simulink library "MISSILE_GUIDANCE_LIB2"  (R2025b)
settings: Solver=VariableStepAuto  StartTime=0.0  StopTime=10.0  RelTol=1e-3
undefined symbols (not defined in the file or in its folder): accelerationL0, angularPoseL0, angularRateL0, B2D, Continuous, ddLambda, dLambda, dRange, epsMEAS_D, L02B, Lambda, positionL0, psiDotCmd, psiMeas, Range, rangeDotMEAS_D, rangeMEAS_D, t_go, t_sim, targetEps_D, targetRelPos_B, targetRelPos_D, targetRelPos_L0, targetRelVel_L0, targetValid, thetaDotCmd, thetaMeas, Time, timeOfMeas, velocityL0, wAfterStabTF, wCmd_Rtn
libraries: $bdroot x27, simulink x8, simulink_extras x6, matrix_library x3, Missile_Guidance_LIB x1, ctrlSharedLib x1
(part 1 of 2)
settings Model: Creator=leoni  LastModifiedBy=Leonid
settings RTWCC: GPUComputeCapability=3.5

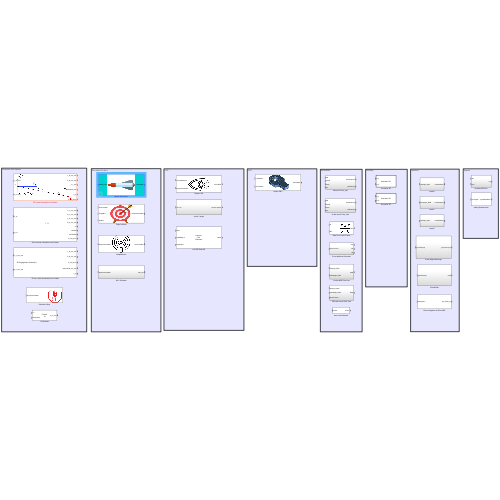
[thumbnail: Simulink's stored preview of the top-level diagram]
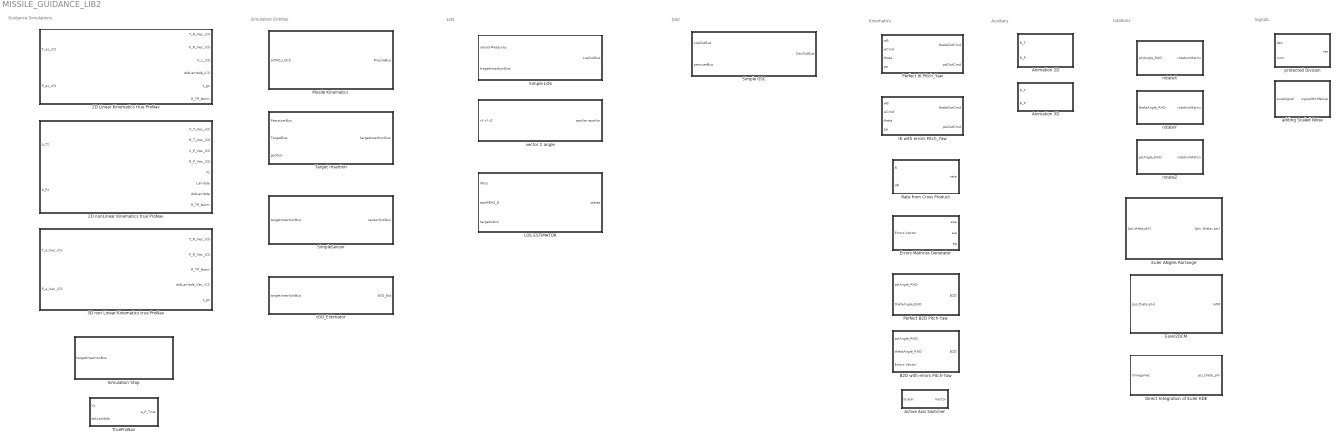
== system MISSILE_GUIDANCE_LIB2 ==
  note: Signals
  note: Auxiliary
  note: LOS
  note: GSC
  note: Simulation Entities
  note: rotations
  note: Kinematics
  note: Guidance Simulations
  2D Linear Kinematics true ProNav : Subsystem  mask{T_Vx0_iCS=-300, T_R0_Vec_iCS=[13000;0], P_Vx0_pCS=1000, P_R0_Vec_iCS=[0;0], HE=-20}
      mask prompts: T_Vx0_iCS "Target Horizontal Velocity [m/s]"; T_R0_Vec_iCS "Initial Target Position Vector [m]"; P_Vx0_pCS "Persuer velocity [m/s]"; P_R0_Vec_iCS "Initial Persuer Position Vector [m]"; HE "Persuer Heading Error Angle [deg]"
      mask DialogControl TargetGroup Prompt: Target Properties
      mask DialogControl PersuerGroup Prompt: Persuer Properties
      mask Display: image('Linearized 2D proNav Guidance.png');
  2D nonLinear Kinematics true ProNav : Subsystem  mask{V_T=300, R_Tx_0=1000, R_Tz_0=10, beta_0=rad2deg(10e-3), V_P=0, R_Px_0=0, R_Pz_0=0, gamma_0=0}
      mask prompts: V_T "Target Velocity [m/s]"; R_Tx_0 "Initial Target Position x [m]"; R_Tz_0 "Initial Target Position z [m]"; beta_0 "Initial Target Angle[deg]"; V_P "Persuer Velocity [m/s]"; R_Px_0 "Initial Pursuer Position x [m]"; R_Pz_0 "Initial Pursuer Position z [m]"; gamma_0 "Initial Pursuer Flight Path Angle[deg]"
      mask DialogControl TargetGroup Prompt: Target Properties
      mask DialogControl PursuerGroup Prompt: Pursuer properties
      mask Display: image('Collision_Course_Kinematics_2D.jpg');
  3D non Linear Kinematics true ProNav : Subsystem  mask{T_V0_Vec_iCS=[300*cos(10e-3);0;300*sin(10e-3)], T_R0_Vec_iCS=[-1000;0;0], P_V0_Vec_iCS=[0;0;0], P_R0_Vec_iCS=[0;0;0]}
      mask prompts: T_V0_Vec_iCS "Target Initial Velocity Vector [m/s]"; T_R0_Vec_iCS "Initial Target Position Vector [m]"; P_V0_Vec_iCS "Persuer Initial Velocity vector [m/s]"; P_R0_Vec_iCS "Initial Persuer Position Vector [m]"
      mask init:
      | if ~exist('Missile_Guidance_Bus_Load_Ok', 'var')
      | run Missile_Guidance_Buses.m
      | assignin('base', 'Missile_Guidance_Bus_Load_Ok', true);
      | fprintf('---- Missile Guidance Buses Loaded Ok ---- \n');
      | 
      | end
      mask DialogControl TargetGroup Prompt: Target Properties
      mask DialogControl PersuerGroup Prompt: Persuer Properties
      mask Display: text(0.05, 0.5, '3D Engagement Kinematics');
  Active Axis Switcher : Subsystem  mask{activeAxis=P motion}
      mask prompts: activeAxis "Base Sine Wave Selector"
      mask TypeOptions activeAxis: P motion | Q motion | R motion
  Animation 2D : MATLAB Function  TreatAsAtomicUnit=on  SystemSampleTime=0.1  mask{xlimVec=[-100 1100], ylimVec=[-20 20]}
      mask prompts: xlimVec "xlim [m]"; ylimVec "ylim [m]"
      mask init:
      | figure('Name','Simulation')
      |     close all;
      |     clf;
      |     plot([],[]); hold on;
      | 
      | 
      |     xlim(xlimVec)
      |     ylim(ylimVec)
      |     % axis equal
      |     grid minor
      |     xlabel('Xaxis [m]')
      |     ylabel('Zaxis [m]')
  Animation 3D : MATLAB Function  TreatAsAtomicUnit=on  SystemSampleTime=0.1  mask{xlimVec=[-1000 20], ylimVec=[-10 10], zlimVec=[-20 20]}
      mask prompts: xlimVec "xlim [m]"; ylimVec "ylim [m]"; zlimVec "zlim [m]"
      mask init:
      | figure('Name','Simulation3D')
      |     close all;
      |     clf;
      |     plot3([0],[0],[0]); hold on;
      | 
      | 
      |     xlim(xlimVec)
      |     ylim(ylimVec)
      |     zlim(zlimVec)
      |     % axis equal
      |     grid minor
      |     xlabel('Xaxis [m]')
      |     ylabel('Yaxis [m]')
      |     zlabel('Zaxis [m]')
  B2D with errors Pitch-Yaw : Subsystem
  Direct Integration of Euler KDE : Subsystem  mask{psi0_theta0_phi0=[0;0;0]}
      mask prompts: psi0_theta0_phi0 "Initial Pose Angles [psi0;theta0;phi0] [deg]"
      mask DialogControl ic1 Prompt: Initial Conditions
  Errors Matrices Generator : Subsystem
  Euler ANgles Rarrange : Subsystem
  Euler2DCM : Subsystem
  IK with errors Pitch_Yaw : Subsystem
  LOS ESTIMATOR : Subsystem  mask{Q=0.1, R=0.1}
      mask prompts: Q "Q - value"; R "R - value"
      mask DialogControl ParameterGroupVar Prompt: Esimator Parameters
      mask Display: disp('Lambda \n Dot \n Estimator');
  Missile Kinematics : Subsystem  mask{psi0_theta0_phi0=[0;0;0], vX0=0, r0=[0;0;0], tau_X=0, tau_YZ=0}
      mask prompts: psi0_theta0_phi0 "Initial [psi0;theta0;phi0] Angles [deg]"; vX0 "Initial Velocity missile X [m/s]"; r0 "Initial Position L0 [m]"; tau_X "Longitudinal time constant [s]"; tau_YZ "Lateral time constant [s]"
      mask DialogControl ParameterGroupVar Prompt: Initial Conditions
      mask DialogControl Container3 Prompt: Psuedo Pilot
      mask Display: image('missile.png');
  Perfect B2D Pitch-Yaw : Subsystem
  Perfect IK Pitch_Yaw : Subsystem
  Rate from Cross Product : Subsystem
      mask Display: image('Rate_From_Cross_Product.png');
  Simple GSC : Subsystem  mask{theta0=0, psi0=0, fRATE=0, zetaRATE=0, f_clock_GSC=1800, enErrors=on, errorsVec=zeros(9,1), Jo_kgmm=0, Ji_kgmm=0, Icmd_MAX=0, Kt_mNm=0}
      mask prompts: theta0 "Initial Pitch Angle [deg]"; psi0 "Initial yaw Angle [deg]"; fRATE "Rate Controller fBW [Hz]"; zetaRATE "Rate Controller Zeta"; f_clock_GSC "GSC Working Freq [Hz]"; enErrors "Enable Errors"; errorsVec "Errors Vector - X (terms)"; Jo_kgmm "Outer Inertia [kgmm^2]"; Ji_kgmm "Inner Inertia [kgmm^2]"; Icmd_MAX "Current Limit [A]"; Kt_mNm "Motor Constant [mNm/A]"
      mask DialogControl ParameterGroupVar Prompt: Initial Conditions
      mask DialogControl Container3 Prompt: Rate Controller
      mask DialogControl Container4 Prompt: RT parameters
      mask DialogControl Container5 Prompt: Installation Errors
      mask DialogControl Container6 Prompt: Mass Params
      mask DialogControl Container7 Prompt: Current Params
      mask Display: image('GIMBALS.png');
  Simple LOS : Subsystem  mask{kLOS=0, f_clock_LOS=600, perfectPoint=on, perfectTrack=on}
      mask prompts: kLOS "Track Loop Gain"; f_clock_LOS "Los Working Freq [Hz]"; perfectPoint "Is Perfect Point Mode ?"; perfectTrack "Is Perfect Tack Mode ?"
      mask DialogControl ParameterGroupVar Prompt: Controllers
      mask DialogControl Container3 Prompt: RT
      mask DialogControl Container4 Prompt: Assumptions
      mask Display: image('LOS.png');
  SimpleSensor : Subsystem  mask{halfFov=0, epsNoise=0, rangeNoise=0, rangeDotNoise=0, f_clock_SENS=100, tLatency=10}
      mask prompts: halfFov "Half Sensors FOV [deg]"; epsNoise "Epsilon Noise [rad]"; rangeNoise "Range Noise [m]"; rangeDotNoise "Dopler Noise [m/s]"; f_clock_SENS "Reporting Freq. [Hz]"; tLatency "Reporting Latency [ms]"
      mask DialogControl ParameterGroupVar Prompt: Sensor Parameters
      mask DialogControl Container3 Prompt: RT Parameters
      mask Display: image('Sensor.png');
  Simulation Stop : Subsystem  mask{tGO_Limit=0}
      mask prompts: tGO_Limit "Maximum TGO Value [s]"
      mask Display: image('STOP.png');
  Target Insertion : Subsystem
      mask Display: image('Target.png');
  TrueProNav : Subsystem  mask{N=3}
      mask prompts: N "ProNav Coefficient - N"
      mask Display: disp('ProNav\n N');
  adding Scaled Noise : Subsystem  mask{noiseProc=0}
      mask prompts: noiseProc "Noise [%] from Signal"
  protected Division : Subsystem
  rotateX : Subsystem
  rotateY : Subsystem
  rotateZ : Subsystem
  tGO_Estimator : Subsystem
  vector 2 angle : Subsystem

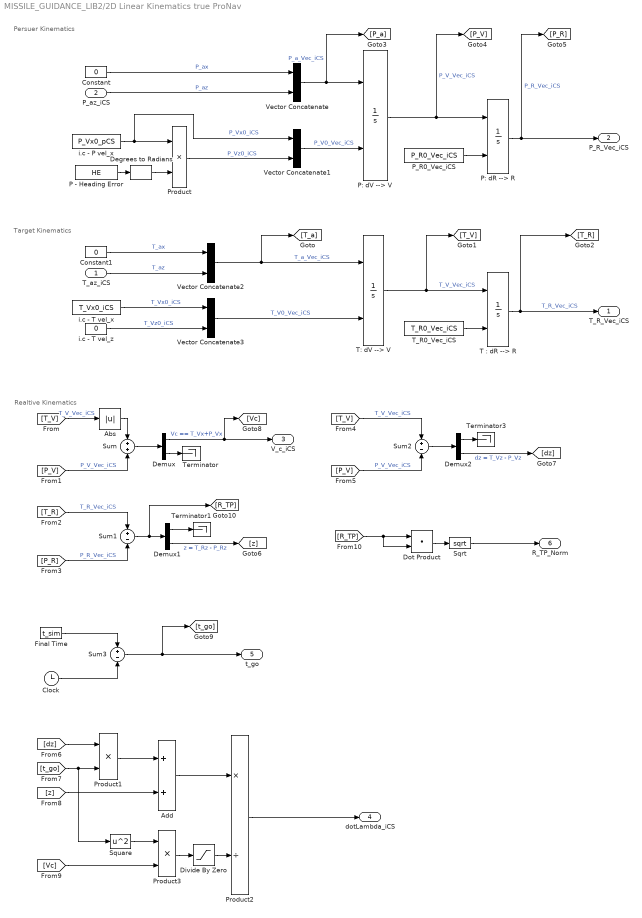
== system MISSILE_GUIDANCE_LIB2/2D Linear Kinematics true ProNav ==
  note: Persuer Kinematics
  note: Target Kinematics
  note: Realtive Kinematics
  T_az_iCS : Inport
  P_az_iCS : Inport  Port=2
  Abs : Abs  SaturateOnIntegerOverflow=off
  Add : Sum
  Clock : Clock
  Constant : Constant  Value=0
  Constant1 : Constant  Value=0
  Degrees to Radians : simulink_extras/Transformations/Degrees to Radians
  Demux : Demux  Outputs=2
  Demux1 : Demux  Outputs=2
  Demux2 : Demux  Outputs=2
  Divide By Zero : Saturate  UpperLimit=Inf  LowerLimit=1e-9
  Dot Product : DotProduct  OutDataTypeStr=Inherit: Inherit via internal rule
  Final Time : Constant  Value=t_sim
  P - Heading Error : Constant  Value=HE
  P: dR --> R : Integrator  InitialConditionSource=external
  P: dV --> V : Integrator  InitialConditionSource=external
  P_R0_Vec_iCS : Constant  Value=P_R0_Vec_iCS
  Product : Product
  Product1 : Product
  Product2 : Product  Inputs=*/
  Product3 : Product
  Sqrt : Sqrt
  Square : Math  Operator=square
  Sum : Sum  Inputs=+|+
  Sum1 : Sum  Inputs=+|-
  Sum2 : Sum  Inputs=+|-
  Sum3 : Sum  Inputs=+|-
  "T : dR --> R" : Integrator  InitialConditionSource=external
  T: dV --> V : Integrator  InitialConditionSource=external
  T_R0_Vec_iCS : Constant  Value=T_R0_Vec_iCS
  Terminator : Terminator
  Terminator1 : Terminator
  Terminator3 : Terminator
  Vector Concatenate{,1..3} (4 alike) : Concatenate  Mode=Multidimensional array
  i.c - P vel_x : Constant  Value=P_Vx0_pCS
  i.c - T vel_x : Constant  Value=T_Vx0_iCS
  i.c - T vel_z : Constant  Value=0
  T_R_Vec_iCS : Outport
  P_R_Vec_iCS : Outport  Port=2
  V_c_iCS : Outport  Port=3
  dotLambda_iCS : Outport  Port=4
  t_go : Outport  Port=5
  R_TP_Norm : Outport  Port=6
  wires:
  Divide By Zero/1 -> Product2/2
  Abs/1 -> Sum/1
  Sqrt/1 -> R_TP_Norm/1
  Dot Product/1 -> Sqrt/1
  [R_TP] -> Dot Product/1, Dot Product/2
  Product2/1 -> dotLambda_iCS/1
  Product3/1 -> Divide By Zero/1
  Square/1 -> Product3/1
  [Vc] -> Product3/2
  Add/1 -> Product2/1
  [z] -> Add/2
  Product1/1 -> Add/1
  [dz] -> Product1/1
  [t_go] -> Product1/2, Square/1
  Sum3/1 -> [t_go], t_go/1
  Final Time/1 -> Sum3/1
  Clock/1 -> Sum3/2
  [P_V] -> Sum2/2  "P_V_Vec_iCS"
  [T_V] -> Sum2/1  "T_V_Vec_iCS"
  Sum2/1 -> Demux2/1
  Demux2/1 -> Terminator3/1
  Demux2/2 -> [dz]  "dz = T_Vz - P_Vz"
  Demux1/2 -> [z]  "z = T_Rz - P_Rz"
  Demux1/1 -> Terminator1/1
  Sum1/1 -> Demux1/1, [R_TP]
  [P_R] -> Sum1/2  "P_R_Vec_iCS"
  [T_R] -> Sum1/1  "T_R_Vec_iCS"
  Demux/1 -> V_c_iCS/1, [Vc]  "Vc == T_Vx+P_Vx"
  Demux/2 -> Terminator/1
  Sum/1 -> Demux/1
  [P_V] -> Sum/2  "P_V_Vec_iCS"
  [T_V] -> Abs/1  "T_V_Vec_iCS"
  "T : dR --> R"/1 -> T_R_Vec_iCS/1, [T_R]  "T_R_Vec_iCS"
  T_R0_Vec_iCS/1 -> "T : dR --> R"/2
  Degrees to Radians/1 -> Product/2
  T: dV --> V/1 -> "T : dR --> R"/1, [T_V]  "T_V_Vec_iCS"
  Vector Concatenate3/1 -> T: dV --> V/2  "T_V0_Vec_iCS"
  i.c - T vel_z/1 -> Vector Concatenate3/2  "T_Vz0_iCS"
  i.c - T vel_x/1 -> Vector Concatenate3/1  "T_Vx0_iCS"
  Vector Concatenate2/1 -> T: dV --> V/1, [T_a]  "T_a_Vec_iCS"
  Constant1/1 -> Vector Concatenate2/1  "T_ax"
  P: dR --> R/1 -> P_R_Vec_iCS/1, [P_R]  "P_R_Vec_iCS"
  Vector Concatenate1/1 -> P: dV --> V/2  "P_V0_Vec_iCS"
  Vector Concatenate/1 -> P: dV --> V/1, [P_a]  "P_a_Vec_iCS"
  Constant/1 -> Vector Concatenate/1  "P_ax"
  Product/1 -> Vector Concatenate1/2  "P_Vz0_iCS"
  P - Heading Error/1 -> Degrees to Radians/1
  P_R0_Vec_iCS/1 -> P: dR --> R/2
  P: dV --> V/1 -> P: dR --> R/1, [P_V]  "P_V_Vec_iCS"
  i.c - P vel_x/1 -> Product/1, Vector Concatenate1/1  "P_Vx0_iCS"
  P_az_iCS/1 -> Vector Concatenate/2  "P_az"
  T_az_iCS/1 -> Vector Concatenate2/2  "T_az"

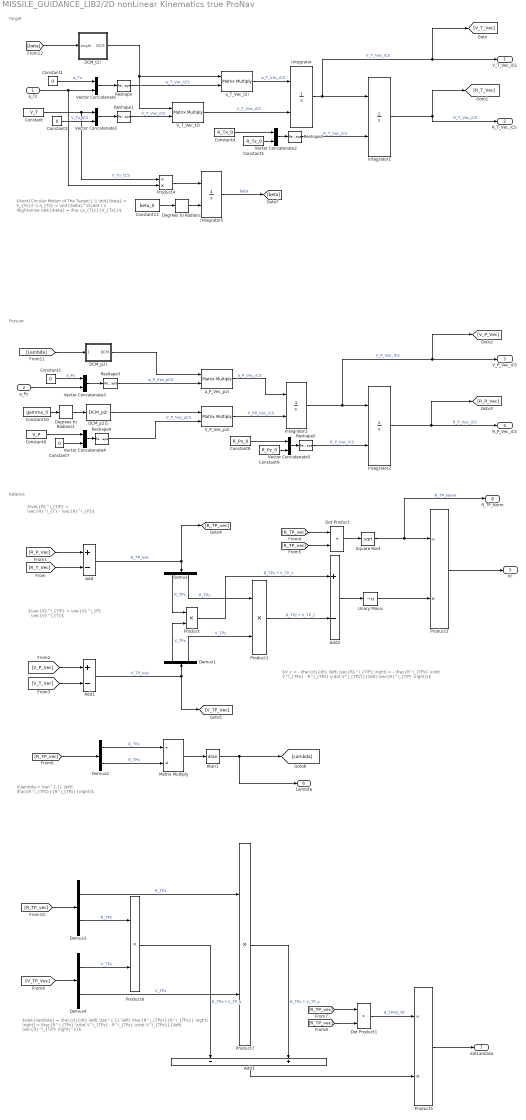
== system MISSILE_GUIDANCE_LIB2/2D nonLinear Kinematics true ProNav ==
  note: $\dot{\lambda} = \frac{d}{dt} \left[ \tan^{-1} \left( \frac{R^i_{TPz}}{R^i_{TPx}} \right) \right] = \frac{R^i_{TPx} \cdot V^i_{TPz} - R^i_{TPz} \cdot V^i_{TPx}}{\left| \vec{R}^i_{T/P} \right|^2}$
  note: $\vec{V}^i_{T/P} = \vec{V}^i_{P} - \vec{V}^i_{T}$
  note: Persuer
  note: Target
  note: Relative
  note: $\vec{R}^i_{T/P} = \vec{R}^i_{T} - \vec{R}^i_{P}$
  note: $V_c = - \frac{d}{dt} \left| \vec{R}^i_{T/P} \right| = - \frac{R^i_{TPx} \cdot V^i_{TPx} - R^i_{TPz} \cdot V^i_{TPz}}{\left| \vec{R}^i_{T/P} \right|}$
  note: $\lambda = \tan^{-1} \left( \frac{R^i_{TPz}}{R^i_{TPx}}\right)$
  note: $\text{Circular Motion of The Target:} \\ \dot{\beta} = V_{Tx}/r \\ a_{Tz} = \dot{\beta}^2\cdot r \\ \Rightarrow \dot{\beta} = \frac{a_{Tz}}{V_{Tx}}$
  a_Tz : Inport
  a_Pz : Inport  Port=2
  Add : Sum  Inputs=+-
  Add1 : Sum  Inputs=+-
  Add2 : Sum  Inputs=+-
  Add3 : Sum  Inputs=-+
  Atan1 : Trigonometry  Operator=atan
  Constant : Constant  Value=V_T
  Constant{1..3,7} (4 alike) : Constant  Value=0
  Constant10 : Constant  Value=gamma_0
  Constant11 : Constant  Value=beta_0
  Constant4 : Constant  Value=R_Tx_0
  Constant5 : Constant  Value=R_Tz_0
  Constant6 : Constant  Value=V_P
  Constant8 : Constant  Value=R_Px_0
  Constant9 : Constant  Value=R_Pz_0
  DCM_p2i : Subsystem
  DCM_p2i1 : Missile_Guidance_LIB/2D nonLinear Kinematics true ProNav/DCM_p2i  SystemSampleTime=-1  VariantActivationTime=update diagram  AllowFlexibleInterface=on  Latency=0  AutoFrameSizeCalculation=off
  DCM_t2i : Subsystem
  Degrees to Radians : simulink_extras/Transformations/Degrees to Radians
  Degrees to Radians1 : simulink_extras/Transformations/Degrees to Radians
  Demux{,1..4} (5 alike) : Demux  Outputs=2
  Dot Product : DotProduct  OutDataTypeStr=Inherit: Inherit via internal rule
  Dot Product1 : DotProduct  OutDataTypeStr=Inherit: Inherit via internal rule
  Integrator{,1..3,5} (5 alike) : Integrator  InitialConditionSource=external
  Matrix Multiply : Product  Inputs=/*
  Product{,1,6..7} (4 alike) : Product
  Product2 : Product  Inputs=/*
  Product4 : Product  Inputs=/*
  Product5 : Product  Inputs=/*
  Reshape{,1..5} (6 alike) : Reshape  OutputDimensionality=Column vector (2-D)
  Square Root : Sqrt
  Unary Minus : UnaryMinus
  V_P_Vec_p2i : Product  Multiplication=Matrix(*)
  V_T_Vec_t2i : Product  Multiplication=Matrix(*)
  Vector Concatenate{,1..5} (6 alike) : Concatenate
  a_P_Vec_p2i : Product  Multiplication=Matrix(*)
  a_T_Vec_t2i : Product  Multiplication=Matrix(*)
  V_T_Vec_iCS : Outport
  R_T_Vec_iCS : Outport  Port=2
  V_P_Vec_iCS : Outport  Port=3
  R_P_Vec_iCS : Outport  Port=4
  Vc : Outport  Port=5
  Lambda : Outport  Port=6
  dotLambda : Outport  Port=7
  R_TP_Norm : Outport  Port=8
  wires:
  Atan1/1 -> [Lambda], Lambda/1
  Matrix Multiply/1 -> Atan1/1
  Degrees to Radians1/1 -> DCM_p2i1/1
  DCM_p2i1/1 -> V_P_Vec_p2i/1
  Constant10/1 -> Degrees to Radians1/1
  V_P_Vec_p2i/1 -> Integrator2/2  "V_P0_Vec_iCS"
  Degrees to Radians/1 -> Integrator5/2
  V_T_Vec_t2i/1 -> Integrator/2  "V_T_Vec_iCS"
  Integrator5/1 -> [beta]  "beta"
  Constant11/1 -> Degrees to Radians/1
  Product4/1 -> Integrator5/1
  Product7/1 -> Add3/2  "R_TPx * V_TP_z"
  Product6/1 -> Add3/1  "R_TPz * V_TP_x"
  [R_TP_vec] -> Demux3/1
  [V_TP_Vec] -> Demux4/1
  Demux4/1 -> Product6/2  "V_TPx"
  Demux3/2 -> Product6/1  "R_TPz"
  Demux3/1 -> Product7/1  "R_TPx"
  Demux4/2 -> Product7/2  "V_TPz"
  Product5/1 -> dotLambda/1
  Dot Product1/1 -> Product5/1  "R_TP*R_TP"
  [R_TP_vec] -> Dot Product1/2
  [R_TP_vec] -> Dot Product1/1
  Add3/1 -> Product5/2
  Demux2/2 -> Matrix Multiply/2  "R_TPz"
  Demux2/1 -> Matrix Multiply/1  "R_TPx"
  [R_TP_vec] -> Demux2/1
  Product2/1 -> Vc/1
  Square Root/1 -> Product2/1, R_TP_Norm/1  "R_TP_Norm"
  Dot Product/1 -> Square Root/1
  [R_TP_vec] -> Dot Product/2
  [R_TP_vec] -> Dot Product/1
  Unary Minus/1 -> Product2/2
  Add2/1 -> Unary Minus/1
  Product1/1 -> Add2/2  "R_TPz * V_TP_z"
  Product/1 -> Add2/1  "R_TPx * V_TP_x"
  Demux1/2 -> Product1/2  "V_TPz"
  Demux1/1 -> Product/2  "V_TPx"
  Demux/1 -> Product/1  "R_TPx"
  Demux/2 -> Product1/1  "R_TPz"
  Add1/1 -> Demux1/1, [V_TP_Vec]  "V_TP_Vec"
  [V_T_Vec] -> Add1/2
  [V_P_Vec] -> Add1/1
  Add/1 -> Demux/1, [R_TP_vec]  "R_TP_Vec"
  [R_T_Vec] -> Add/2
  [R_P_Vec] -> Add/1
  Integrator3/1 -> R_P_Vec_iCS/1, [R_P_Vec]  "R_P_Vec_iCS"
  Reshape5/1 -> Integrator3/2  "R_P_Vec_iCS"
  Vector Concatenate5/1 -> Reshape5/1
  Constant8/1 -> Vector Concatenate5/1
  Constant9/1 -> Vector Concatenate5/2
  Integrator2/1 -> Integrator3/1, V_P_Vec_iCS/1, [V_P_Vec]  "V_P_Vec_iCS"
  Constant6/1 -> Vector Concatenate4/1
  Constant7/1 -> Vector Concatenate4/2
  Vector Concatenate4/1 -> Reshape4/1
  Reshape4/1 -> V_P_Vec_p2i/2  "V_P_Vec_pCS"
  a_P_Vec_p2i/1 -> Integrator2/1  "a_P_Vec_iCS"
  Vector Concatenate3/1 -> Reshape3/1
  a_Pz/1 -> Vector Concatenate3/2
  Constant2/1 -> Vector Concatenate3/1  "a_Px"
  Reshape3/1 -> a_P_Vec_p2i/2  "a_P_Vec_pCS"
  DCM_p2i/1(DCM) -> a_P_Vec_p2i/1
  [Lambda] -> DCM_p2i/1(angle)
  Constant5/1 -> Vector Concatenate2/2
  Constant4/1 -> Vector Concatenate2/1
  Vector Concatenate2/1 -> Reshape2/1
  Reshape2/1 -> Integrator1/2  "R_T_Vec_iCS"
  Integrator1/1 -> [R_T_Vec], R_T_Vec_iCS/1  "R_T_Vec_iCS"
  Integrator/1 -> Integrator1/1, V_T_Vec_iCS/1, [V_T_Vec]  "V_T_Vec_iCS"
  Reshape1/1 -> V_T_Vec_t2i/2  "V_T_Vec_iCS"
  Vector Concatenate1/1 -> Reshape1/1
  Constant3/1 -> Vector Concatenate1/2  "V_Tz_tCS"
  Constant/1 -> Vector Concatenate1/1, Product4/1  "V_Tx_tCS"
  a_T_Vec_t2i/1 -> Integrator/1  "a_T_Vec_iCS"
  Reshape/1 -> a_T_Vec_t2i/2  "a_T_Vec_tCS"
  Vector Concatenate/1 -> Reshape/1
  Constant1/1 -> Vector Concatenate/1  "a_Tx"
  DCM_t2i/1(DCM) -> a_T_Vec_t2i/1, V_T_Vec_t2i/1
  [beta] -> DCM_t2i/1(angle)
  a_Tz/1 -> Product4/2, Vector Concatenate/2

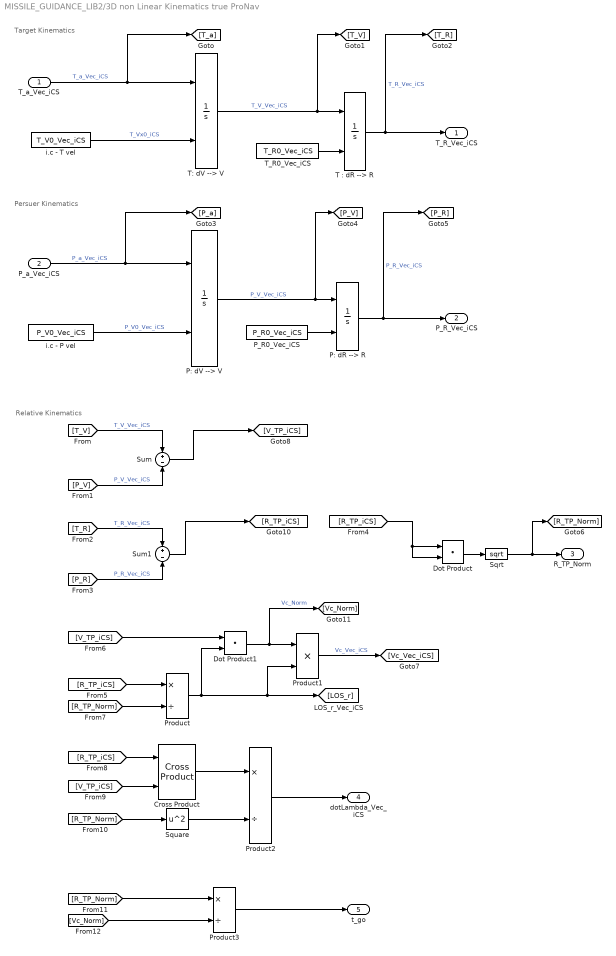
== system MISSILE_GUIDANCE_LIB2/3D non Linear Kinematics true ProNav ==
  note: Target Kinematics
  note: Persuer Kinematics
  note: Relative Kinematics
  T_a_Vec_iCS : Inport  PortDimensions=[3;1]
  P_a_Vec_iCS : Inport  Port=2  PortDimensions=[3;1]
  Cross Product : matrix_library/Cross Product
  Dot Product : DotProduct  OutDataTypeStr=Inherit: Inherit via internal rule
  Dot Product1 : DotProduct  OutDataTypeStr=Inherit: Inherit via internal rule
  P: dR --> R : Integrator  InitialConditionSource=external
  P: dV --> V : Integrator  InitialConditionSource=external
  P_R0_Vec_iCS : Constant  Value=P_R0_Vec_iCS
  Product : Product  Inputs=*/
  Product1 : Product  Inputs=**
  Product2 : Product  Inputs=*/
  Product3 : Product  Inputs=*/
  Sqrt : Sqrt
  Square : Math  Operator=square
  Sum : Sum  Inputs=+|-
  Sum1 : Sum  Inputs=+|-
  "T : dR --> R" : Integrator  InitialConditionSource=external
  T: dV --> V : Integrator  InitialConditionSource=external
  T_R0_Vec_iCS : Constant  Value=T_R0_Vec_iCS
  i.c - P vel : Constant  Value=P_V0_Vec_iCS
  i.c - T vel : Constant  Value=T_V0_Vec_iCS
  T_R_Vec_iCS : Outport
  P_R_Vec_iCS : Outport  Port=2
  R_TP_Norm : Outport  Port=3
  dotLambda_Vec_iCS : Outport  Port=4
  t_go : Outport  Port=5
  wires:
  [Vc_Norm] -> Product3/2
  [R_TP_Norm] -> Product3/1
  Product3/1 -> t_go/1
  Product2/1 -> dotLambda_Vec_iCS/1
  Square/1 -> Product2/2
  [R_TP_Norm] -> Square/1
  Cross Product/1 -> Product2/1
  [V_TP_iCS] -> Cross Product/2
  [R_TP_iCS] -> Cross Product/1
  Product1/1 -> [Vc_Vec_iCS]  "Vc_Vec_iCS"
  Dot Product1/1 -> Product1/1, [Vc_Norm]  "Vc_Norm"
  [V_TP_iCS] -> Dot Product1/1
  Product/1 -> [LOS_r], Product1/2, Dot Product1/2
  [R_TP_Norm] -> Product/2
  [R_TP_iCS] -> Product/1
  T_a_Vec_iCS/1 -> T: dV --> V/1, [T_a]  "T_a_Vec_iCS"
  P_a_Vec_iCS/1 -> [P_a], P: dV --> V/1  "P_a_Vec_iCS"
  i.c - P vel/1 -> P: dV --> V/2  "P_V0_Vec_iCS"
  P: dV --> V/1 -> P: dR --> R/1, [P_V]  "P_V_Vec_iCS"
  P_R0_Vec_iCS/1 -> P: dR --> R/2
  P: dR --> R/1 -> [P_R], P_R_Vec_iCS/1  "P_R_Vec_iCS"
  i.c - T vel/1 -> T: dV --> V/2  "T_Vx0_iCS"
  T: dV --> V/1 -> [T_V], "T : dR --> R"/1  "T_V_Vec_iCS"
  T_R0_Vec_iCS/1 -> "T : dR --> R"/2
  "T : dR --> R"/1 -> T_R_Vec_iCS/1, [T_R]  "T_R_Vec_iCS"
  [T_V] -> Sum/1  "T_V_Vec_iCS"
  [P_V] -> Sum/2  "P_V_Vec_iCS"
  Sum/1 -> [V_TP_iCS]
  [T_R] -> Sum1/1  "T_R_Vec_iCS"
  [P_R] -> Sum1/2  "P_R_Vec_iCS"
  Sum1/1 -> [R_TP_iCS]
  [R_TP_iCS] -> Dot Product/2, Dot Product/1
  Dot Product/1 -> Sqrt/1
  Sqrt/1 -> R_TP_Norm/1, [R_TP_Norm]

== system MISSILE_GUIDANCE_LIB2/Active Axis Switcher ==
  Scalar : Inport
  Compare To Constant : simulink/Logic and Bit Operations/Compare To Constant  relop===  const=1  OutDataTypeStr=boolean
  Compare To Constant1 : simulink/Logic and Bit Operations/Compare To Constant  relop===  const=2  OutDataTypeStr=boolean
  Compare To Constant2 : simulink/Logic and Bit Operations/Compare To Constant  relop===  const=3  OutDataTypeStr=boolean
  Constant : Constant  Value=0
  Constant1 : Constant  Value=activeAxis
  Switch : Switch  Criteria=u2 > Threshold  SaturateOnIntegerOverflow=off  InputSameDT=off
  Switch1 : Switch  Criteria=u2 > Threshold  SaturateOnIntegerOverflow=off  InputSameDT=off
  Switch2 : Switch  Criteria=u2 > Threshold  SaturateOnIntegerOverflow=off  InputSameDT=off
  Vector Concatenate : Concatenate  NumInputs=3
  Vector : Outport
  wires:
  Scalar/1 -> [Source]
  Switch1/1 -> Vector Concatenate/2
  Switch/1 -> Vector Concatenate/1
  Switch2/1 -> Vector Concatenate/3
  Constant1/1 -> Compare To Constant1/1, Compare To Constant/1, Compare To Constant2/1
  Compare To Constant/1 -> Switch/2
  [Source] -> Switch2/1, Switch1/1, Switch/1
  Compare To Constant2/1 -> Switch2/2
  Compare To Constant1/1 -> Switch1/2
  Constant/1 -> Switch2/3, Switch1/3, Switch/3
  Vector Concatenate/1 -> Vector/1  "X Y Z"

== system MISSILE_GUIDANCE_LIB2/B2D with errors Pitch-Yaw ==
  note: $\text{Expansion of kinemtics, when relative velocities vectos omitted for clarity} \\ \omega_b^{gCS} = \underbrace{R_Y(eg_2) \cdot R_X(eg_1) \cdot R_Z (eg_3)}_{eg} \cdot R_{\psi}(\psi+\psi_o)\cdot \underbrace{R_z(eia_3) \cdot R_X(eia_1) \cdot R_Y(eia_2)}_{eia} \cdot R_{\theta}(\theta+\theta_o) \cdot \underbrace{R_Y(eoa_2) \cdot R_X(eoa_1) \cdot R_Z(eoa_3)}_{eoa} \cdot \omega_b^{bCS}$
  note: Inputs
  psiAngle_RAD : Inport
  thetaAngle_RAD : Inport  Port=2
  Errors Vector : Inport  Port=3
  B ---> D : Product  Inputs=5  Multiplication=Matrix(*)
  Errors Matrices Generator : $bdroot/Errors Matrices Generator  SystemSampleTime=-1  VariantActivationTime=update diagram  AllowFlexibleInterface=on  Latency=0  AutoFrameSizeCalculation=off
  rotateY : $bdroot/rotateY  SystemSampleTime=-1  VariantActivationTime=update diagram  AllowFlexibleInterface=on  Latency=0  AutoFrameSizeCalculation=off
  rotateZ : $bdroot/rotateZ  SystemSampleTime=-1  VariantActivationTime=update diagram  AllowFlexibleInterface=on  Latency=0  AutoFrameSizeCalculation=off
  B2D : Outport
  wires:
  thetaAngle_RAD/1 -> rotateY/1
  psiAngle_RAD/1 -> rotateZ/1
  rotateY/1 -> B ---> D/4  "Ro"
  B ---> D/1 -> B2D/1
  rotateZ/1 -> B ---> D/2  "Ri"
  Errors Vector/1 -> Errors Matrices Generator/1  "eoa_1 eoa_2 eoa_3 eia_1 eia_2 eia_3 eg_1 eg_2 eg_3"
  Errors Matrices Generator/1 -> [eoa]
  Errors Matrices Generator/2 -> [eia]
  Errors Matrices Generator/3 -> [eg]
  [eoa] -> B ---> D/5  "Imu2og"
  [eia] -> B ---> D/3  "ig2og"
  [eg] -> B ---> D/1  "ig2gyro"

== system MISSILE_GUIDANCE_LIB2/Direct Integration of Euler KDE ==
  note: 3-2-1 Euler Angle Kinematic Differential Equation
  OmegaVec : Inport
  Degrees to Radians : simulink_extras/Transformations/Degrees to Radians
  Integrator : Integrator  InitialConditionSource=external  InitialCondition=[0;0;0]
  MATLAB Function : MATLAB Function  TreatAsAtomicUnit=on
  MatrixMultiply : Product  Multiplication=Matrix(*)
  initial Pose [deg] : Constant  Value=psi0_theta0_phi0
  psi_theta_phi : Outport
  wires:
  OmegaVec/1 -> MatrixMultiply/2  "omegaVec"
  MATLAB Function/1(A) -> MatrixMultiply/1  "A Matrix"
  MatrixMultiply/1 -> Integrator/1  "der_poseVec"
  Integrator/1 -> MATLAB Function/1(posVec), psi_theta_phi/1
  initial Pose [deg]/1 -> Degrees to Radians/1
  Degrees to Radians/1 -> Integrator/2

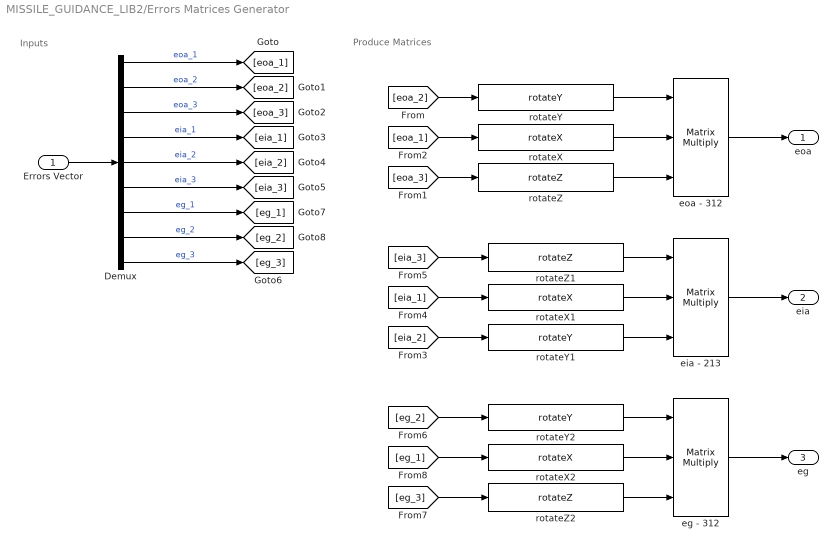
== system MISSILE_GUIDANCE_LIB2/Errors Matrices Generator ==
  note: Produce Matrices
  note: Inputs
  "Errors Vector " : Inport
  Demux : Demux  Outputs=9
  eg - 312 : Product  Inputs=3  Multiplication=Matrix(*)
  eia - 213 : Product  Inputs=3  Multiplication=Matrix(*)
  eoa - 312 : Product  Inputs=3  Multiplication=Matrix(*)
  rotateX : $bdroot/rotateX  SystemSampleTime=-1  VariantActivationTime=update diagram  AllowFlexibleInterface=on  Latency=0  AutoFrameSizeCalculation=off
  rotateX1 : $bdroot/rotateX  SystemSampleTime=-1  VariantActivationTime=update diagram  AllowFlexibleInterface=on  Latency=0  AutoFrameSizeCalculation=off
  rotateX2 : $bdroot/rotateX  SystemSampleTime=-1  VariantActivationTime=update diagram  AllowFlexibleInterface=on  Latency=0  AutoFrameSizeCalculation=off
  rotateY : $bdroot/rotateY  SystemSampleTime=-1  VariantActivationTime=update diagram  AllowFlexibleInterface=on  Latency=0  AutoFrameSizeCalculation=off
  rotateY1 : $bdroot/rotateY  SystemSampleTime=-1  VariantActivationTime=update diagram  AllowFlexibleInterface=on  Latency=0  AutoFrameSizeCalculation=off
  rotateY2 : $bdroot/rotateY  SystemSampleTime=-1  VariantActivationTime=update diagram  AllowFlexibleInterface=on  Latency=0  AutoFrameSizeCalculation=off
  rotateZ : $bdroot/rotateZ  SystemSampleTime=-1  VariantActivationTime=update diagram  AllowFlexibleInterface=on  Latency=0  AutoFrameSizeCalculation=off
  rotateZ1 : $bdroot/rotateZ  SystemSampleTime=-1  VariantActivationTime=update diagram  AllowFlexibleInterface=on  Latency=0  AutoFrameSizeCalculation=off
  rotateZ2 : $bdroot/rotateZ  SystemSampleTime=-1  VariantActivationTime=update diagram  AllowFlexibleInterface=on  Latency=0  AutoFrameSizeCalculation=off
  eoa : Outport
  eia : Outport  Port=2
  eg : Outport  Port=3
  wires:
  "Errors Vector "/1 -> Demux/1
  Demux/1 -> [eoa_1]  "eoa_1"
  Demux/2 -> [eoa_2]  "eoa_2"
  Demux/3 -> [eoa_3]  "eoa_3"
  Demux/4 -> [eia_1]  "eia_1"
  Demux/5 -> [eia_2]  "eia_2"
  Demux/6 -> [eia_3]  "eia_3"
  Demux/7 -> [eg_1]  "eg_1"
  Demux/8 -> [eg_2]  "eg_2"
  Demux/9 -> [eg_3]  "eg_3"
  rotateZ/1 -> eoa - 312/3
  rotateX/1 -> eoa - 312/2
  rotateY/1 -> eoa - 312/1
  [eoa_2] -> rotateY/1
  [eoa_3] -> rotateZ/1
  [eoa_1] -> rotateX/1
  eoa - 312/1 -> eoa/1
  rotateY1/1 -> eia - 213/3
  [eia_2] -> rotateY1/1
  rotateX1/1 -> eia - 213/2
  [eia_1] -> rotateX1/1
  rotateZ1/1 -> eia - 213/1
  [eia_3] -> rotateZ1/1
  eia - 213/1 -> eia/1
  rotateY2/1 -> eg - 312/1
  rotateX2/1 -> eg - 312/2
  rotateZ2/1 -> eg - 312/3
  [eg_1] -> rotateX2/1
  [eg_2] -> rotateY2/1
  [eg_3] -> rotateZ2/1
  eg - 312/1 -> eg/1

== system MISSILE_GUIDANCE_LIB2/Euler ANgles Rarrange ==
  "[psi,theta,phi]" : Inport
  Demux : Demux  Outputs=3
  Mux : Mux  Inputs=3
  Reshape : Reshape  OutputDimensionality=Column vector (2-D)
  "[phi, theta, psi]" : Outport
  wires:
  "[psi,theta,phi]"/1 -> Demux/1
  Mux/1 -> Reshape/1  "[phi, theta, psi]"
  Reshape/1 -> "[phi, theta, psi]"/1
  Demux/2 -> Mux/2
  Demux/3 -> Mux/1
  Demux/1 -> Mux/3

== system MISSILE_GUIDANCE_LIB2/Euler2DCM ==
  "[psi;theta;phi]" : Inport
  eul2rotm : MATLAB Function  TreatAsAtomicUnit=on
  rotM : Outport
  wires:
  eul2rotm/1(y) -> rotM/1
  "[psi;theta;phi]"/1 -> eul2rotm/1(u)

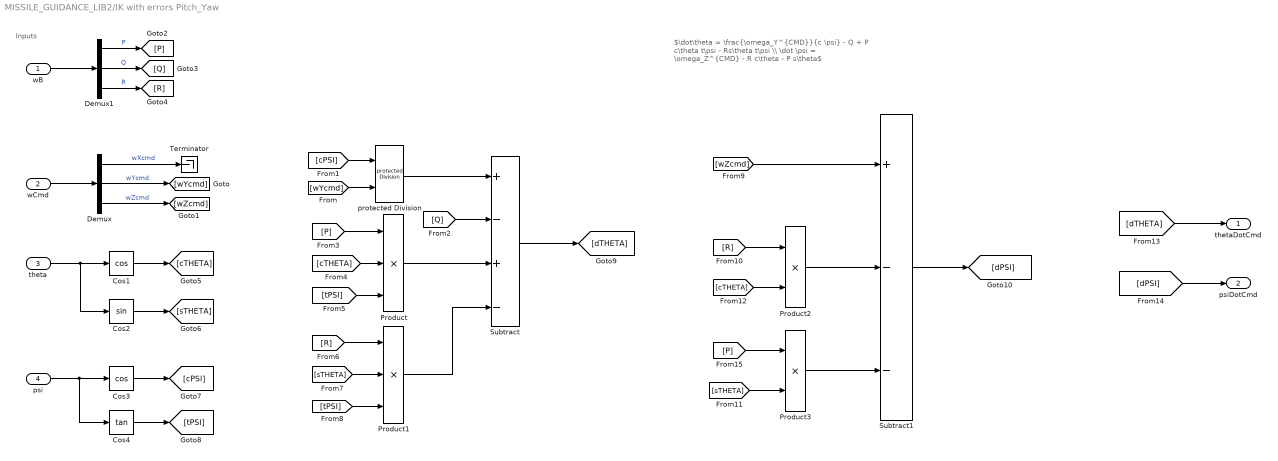
== system MISSILE_GUIDANCE_LIB2/IK with errors Pitch_Yaw ==
  note: Inputs
  note: $\dot\theta = \frac{\omega_Y^{CMD}}{c \psi} - Q + P c\theta t\psi - Rs\theta t\psi \\ \dot \psi = \omega_Z^{CMD} - R c\theta - P s\theta$
  wB : Inport
  wCmd : Inport  Port=2
  theta : Inport  Port=3
  psi : Inport  Port=4
  Cos1 : Trigonometry  Operator=cos
  Cos2 : Trigonometry
  Cos3 : Trigonometry  Operator=cos
  Cos4 : Trigonometry  Operator=tan
  Demux : Demux  Outputs=3
  Demux1 : Demux  Outputs=3
  Product : Product  Inputs=3
  Product1 : Product  Inputs=3
  Product2 : Product
  Product3 : Product
  Subtract : Sum  Inputs=+-+-
  Subtract1 : Sum  Inputs=+--
  Terminator : Terminator
  protected Division : $bdroot/protected Division  SystemSampleTime=-1  VariantActivationTime=update diagram  AllowFlexibleInterface=on  Latency=0  AutoFrameSizeCalculation=off
  thetaDotCmd : Outport
  psiDotCmd : Outport  Port=2
  wires:
  [dPSI] -> psiDotCmd/1
  [dTHETA] -> thetaDotCmd/1
  Subtract1/1 -> [dPSI]
  Product3/1 -> Subtract1/3
  [P] -> Product3/1
  [sTHETA] -> Product3/2
  [cTHETA] -> Product2/2
  Product2/1 -> Subtract1/2
  [R] -> Product2/1
  [wZcmd] -> Subtract1/1
  Subtract/1 -> [dTHETA]
  Product1/1 -> Subtract/4
  [tPSI] -> Product1/3
  [sTHETA] -> Product1/2
  [R] -> Product1/1
  Product/1 -> Subtract/3
  [tPSI] -> Product/3
  [cTHETA] -> Product/2
  [P] -> Product/1
  Cos4/1 -> [tPSI]
  Cos3/1 -> [cPSI]
  psi/1 -> Cos3/1, Cos4/1
  Cos2/1 -> [sTHETA]
  Cos1/1 -> [cTHETA]
  theta/1 -> Cos1/1, Cos2/1
  wCmd/1 -> Demux/1
  Demux/1 -> Terminator/1  "wXcmd"
  Demux/3 -> [wZcmd]  "wZcmd"
  Demux/2 -> [wYcmd]  "wYcmd"
  wB/1 -> Demux1/1
  Demux1/3 -> [R]  "R"
  Demux1/1 -> [P]  "P"
  Demux1/2 -> [Q]  "Q"
  [wYcmd] -> protected Division/2
  [cPSI] -> protected Division/1
  [Q] -> Subtract/2
  protected Division/1 -> Subtract/1

== system MISSILE_GUIDANCE_LIB2/LOS ESTIMATOR ==
  note: $x = \left[ \matrix{ \varepsilon_{VER} \cr \dot \lambda_y \cr \ddot \lambda_y \cr \varepsilon_{HOR} \cr \dot \lambda_z \cr \ddot \lambda_z } \right ]$$
  Wlos : Inport
  epsMEAS_D : Inport  Port=2
  targetValid : Inport  Port=3
  A matrix : MATLAB Function  TreatAsAtomicUnit=on
  B matrix : MATLAB Function  TreatAsAtomicUnit=on
  C matrix : MATLAB Function  TreatAsAtomicUnit=on
  Constant : Constant  Value=zeros(6,1)
  Constant1 : Constant  Value=zeros(6,6)
  D matrix : MATLAB Function  TreatAsAtomicUnit=on
  Demux : Demux  Outputs=3
  Kalman Filter : ctrlSharedLib/Kalman Filter  TimeDomain=Continuous-Time  UseCurrentEstimator=on  ModelSource=Input port  ModelSourceVariable=ss(0.95,1,1,0,1)  A=0.95  B=1  C=1  D=0  NumberOfStates=6  NumberOfInputs=2  NumberOfOutputs=2  InitialEstimateSource=Input port  X0=0  P0=10  UseK=off  UseGH=off  NumberOfProcessNoiseInputs=1  G=1  TimeInvariantG=on  H=0  TimeInvariantH=on  Q=diag([0 0 Q 0 0 Q])  TimeInvariantQ=on  R=R*[1;1]  TimeInvariantR=on  N=0  TimeInvariantN=on  AddInputPort=on  AddEnablePort=on  OutputEstimatedY=off  OutputP=off  Ts=-1
  Mux : Mux  Inputs=2
  Terminator : Terminator
  states : Outport
  wires:
  Wlos/1 -> A matrix/1(Wlos), Demux/1
  targetValid/1 -> Kalman Filter/5
  Kalman Filter/1 -> states/1
  A matrix/1(A) -> Kalman Filter/6
  B matrix/1(B) -> Kalman Filter/7
  Mux/1 -> Kalman Filter/1  "Wy Wz"
  epsMEAS_D/1 -> Kalman Filter/2  "epsVer epsHor"
  C matrix/1(C) -> Kalman Filter/8
  D matrix/1(D) -> Kalman Filter/9
  Constant/1 -> Kalman Filter/3
  Constant1/1 -> Kalman Filter/4
  Demux/2 -> Mux/1
  Demux/3 -> Mux/2
  Demux/1 -> Terminator/1

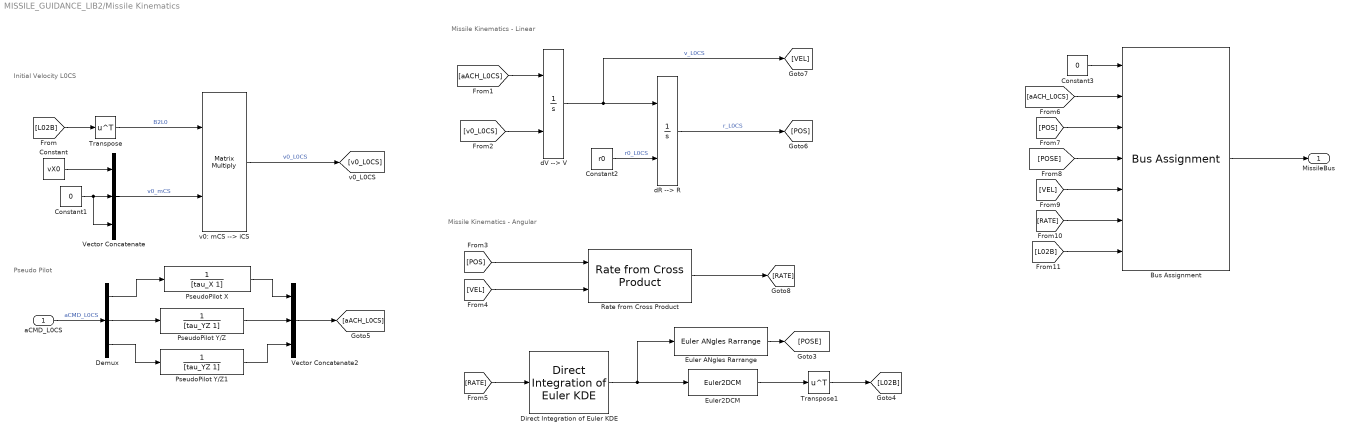
== system MISSILE_GUIDANCE_LIB2/Missile Kinematics ==
  note: Missile Kinematics - Angular
  note: Missile Kinematics - Linear
  note: Pseudo Pilot
  note: Initial Velocity L0CS
  aCMD_L0CS : Inport
  Bus Assignment : BusAssignment  AssignedSignals=accelerationL0,positionL0,angularPoseL0,velocityL0,angularRateL0,L02B
  Constant : Constant  Value=vX0
  Constant1 : Constant  Value=0
  Constant2 : Constant  Value=r0
  Constant3 : Constant  Value=0  OutDataTypeStr=Bus: missileBus
  Demux : Demux  Outputs=3
  Direct Integration of Euler KDE : $bdroot/Direct Integration of Euler KDE  psi0_theta0_phi0=psi0_theta0_phi0
  Euler ANgles Rarrange : $bdroot/Euler ANgles Rarrange  SystemSampleTime=-1  VariantActivationTime=update diagram  EmptyChoice=off  PassThrough=off  PassThroughVariantControl=(default)  EmptyChoiceVariantControl=(default)  AllowFlexibleInterface=on  Latency=0  AutoFrameSizeCalculation=off
  Euler2DCM : $bdroot/Euler2DCM  SystemSampleTime=-1  VariantActivationTime=update diagram  EmptyChoice=off  PassThrough=off  PassThroughVariantControl=(default)  EmptyChoiceVariantControl=(default)  AllowFlexibleInterface=on  Latency=0  AutoFrameSizeCalculation=off
  PseudoPilot X : TransferFcn  Denominator=[tau_X 1]
  PseudoPilot Y/Z : TransferFcn  Denominator=[tau_YZ 1]
  PseudoPilot Y/Z1 : TransferFcn  Denominator=[tau_YZ 1]
  Rate from Cross Product : $bdroot/Rate from Cross Product
  Transpose : Math  Operator=transpose
  Transpose1 : Math  Operator=transpose
  Vector Concatenate : Concatenate  NumInputs=3  Mode=Multidimensional array
  Vector Concatenate2 : Concatenate  NumInputs=3  Mode=Multidimensional array
  dR --> R : Integrator  InitialConditionSource=external
  dV --> V : Integrator  InitialConditionSource=external
  v0: mCS --> iCS : Product  Multiplication=Matrix(*)
  MissileBus : Outport  OutDataTypeStr=Bus: missileBus
  wires:
  Constant/1 -> Vector Concatenate/1
  Constant1/1 -> Vector Concatenate/3, Vector Concatenate/2
  Vector Concatenate/1 -> v0: mCS --> iCS/2  "v0_mCS"
  [L02B] -> Transpose/1
  Transpose/1 -> v0: mCS --> iCS/1  "B2L0"
  v0: mCS --> iCS/1 -> [v0_L0CS]  "v0_L0CS"
  aCMD_L0CS/1 -> Demux/1  "aCMD_L0CS"
  Demux/2 -> PseudoPilot Y/Z/1
  Demux/3 -> PseudoPilot Y/Z1/1
  Demux/1 -> PseudoPilot X/1
  PseudoPilot X/1 -> Vector Concatenate2/1
  PseudoPilot Y/Z/1 -> Vector Concatenate2/2
  Vector Concatenate2/1 -> [aACH_L0CS]
  [aACH_L0CS] -> dV --> V/1
  [v0_L0CS] -> dV --> V/2
  dV --> V/1 -> [VEL], dR --> R/1  "v_L0CS"
  Constant2/1 -> dR --> R/2  "r0_L0CS"
  dR --> R/1 -> [POS]  "r_L0CS"
  [POS] -> Rate from Cross Product/1
  [VEL] -> Rate from Cross Product/2
  Rate from Cross Product/1 -> [RATE]
  Direct Integration of Euler KDE/1 -> Euler2DCM/1, Euler ANgles Rarrange/1
  Euler2DCM/1 -> Transpose1/1
  [RATE] -> Direct Integration of Euler KDE/1
  Constant3/1 -> Bus Assignment/1
  [aACH_L0CS] -> Bus Assignment/2
  [POS] -> Bus Assignment/3
  [POSE] -> Bus Assignment/4
  [VEL] -> Bus Assignment/5
  [RATE] -> Bus Assignment/6
  [L02B] -> Bus Assignment/7
  Bus Assignment/1 -> MissileBus/1
  PseudoPilot Y/Z1/1 -> Vector Concatenate2/3
  Euler ANgles Rarrange/1 -> [POSE]
  Transpose1/1 -> [L02B]

== system MISSILE_GUIDANCE_LIB2/Perfect B2D Pitch-Yaw ==
  psiAngle_RAD : Inport
  thetaAngle_RAD : Inport  Port=2
  Matrix Multiply : Product  Multiplication=Matrix(*)
  rotateY : $bdroot/rotateY  SystemSampleTime=-1  VariantActivationTime=update diagram  AllowFlexibleInterface=on  Latency=0  AutoFrameSizeCalculation=off
  rotateZ : $bdroot/rotateZ  SystemSampleTime=-1  VariantActivationTime=update diagram  AllowFlexibleInterface=on  Latency=0  AutoFrameSizeCalculation=off
  B2D : Outport
  wires:
  rotateZ/1 -> Matrix Multiply/1
  Matrix Multiply/1 -> B2D/1
  rotateY/1 -> Matrix Multiply/2
  psiAngle_RAD/1 -> rotateZ/1
  thetaAngle_RAD/1 -> rotateY/1

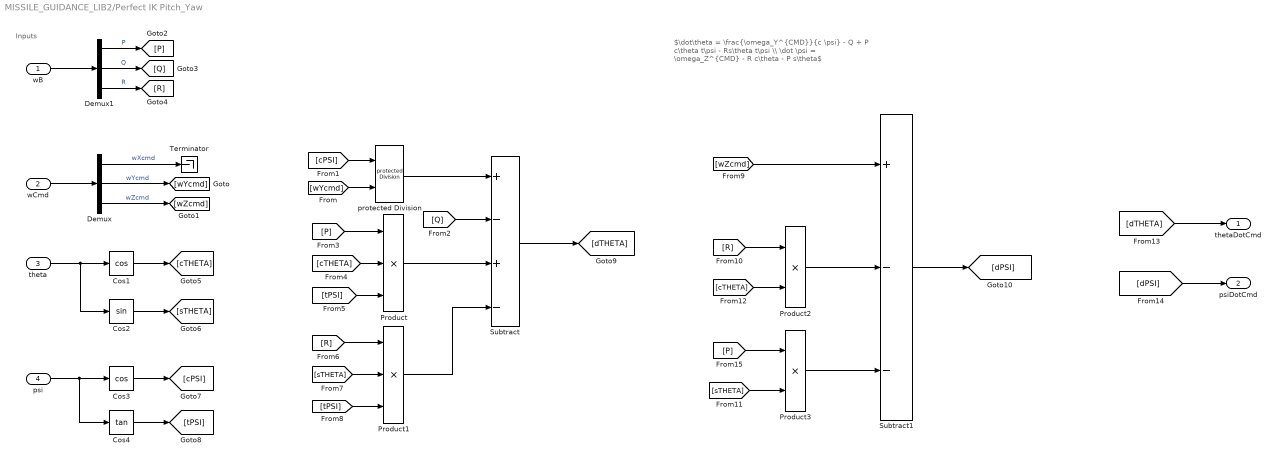
== system MISSILE_GUIDANCE_LIB2/Perfect IK Pitch_Yaw ==
  note: $\dot\theta = \frac{\omega_Y^{CMD}}{c \psi} - Q + P c\theta t\psi - Rs\theta t\psi \\ \dot \psi = \omega_Z^{CMD} - R c\theta - P s\theta$
  note: Inputs
  wB : Inport
  wCmd : Inport  Port=2
  theta : Inport  Port=3
  psi : Inport  Port=4
  Cos1 : Trigonometry  Operator=cos
  Cos2 : Trigonometry
  Cos3 : Trigonometry  Operator=cos
  Cos4 : Trigonometry  Operator=tan
  Demux : Demux  Outputs=3
  Demux1 : Demux  Outputs=3
  Product : Product  Inputs=3
  Product1 : Product  Inputs=3
  Product2 : Product
  Product3 : Product
  Subtract : Sum  Inputs=+-+-
  Subtract1 : Sum  Inputs=+--
  Terminator : Terminator
  protected Division : $bdroot/protected Division  SystemSampleTime=-1  VariantActivationTime=update diagram  AllowFlexibleInterface=on  Latency=0  AutoFrameSizeCalculation=off
  thetaDotCmd : Outport
  psiDotCmd : Outport  Port=2
  wires:
  protected Division/1 -> Subtract/1
  [Q] -> Subtract/2
  [cPSI] -> protected Division/1
  [wYcmd] -> protected Division/2
  Demux1/2 -> [Q]  "Q"
  Demux1/1 -> [P]  "P"
  Demux1/3 -> [R]  "R"
  wB/1 -> Demux1/1
  Demux/2 -> [wYcmd]  "wYcmd"
  Demux/3 -> [wZcmd]  "wZcmd"
  Demux/1 -> Terminator/1  "wXcmd"
  wCmd/1 -> Demux/1
  theta/1 -> Cos2/1, Cos1/1
  Cos1/1 -> [cTHETA]
  Cos2/1 -> [sTHETA]
  psi/1 -> Cos4/1, Cos3/1
  Cos3/1 -> [cPSI]
  Cos4/1 -> [tPSI]
  [P] -> Product/1
  [cTHETA] -> Product/2
  [tPSI] -> Product/3
  Product/1 -> Subtract/3
  [R] -> Product1/1
  [sTHETA] -> Product1/2
  [tPSI] -> Product1/3
  Product1/1 -> Subtract/4
  Subtract/1 -> [dTHETA]
  [wZcmd] -> Subtract1/1
  [R] -> Product2/1
  Product2/1 -> Subtract1/2
  [cTHETA] -> Product2/2
  [sTHETA] -> Product3/2
  [P] -> Product3/1
  Product3/1 -> Subtract1/3
  Subtract1/1 -> [dPSI]
  [dTHETA] -> thetaDotCmd/1
  [dPSI] -> psiDotCmd/1

== system MISSILE_GUIDANCE_LIB2/Rate from Cross Product ==
  R : Inport
  dR : Inport  Port=2
  protected Division1 : $bdroot/protected Division  SystemSampleTime=-1  VariantActivationTime=update diagram  AllowFlexibleInterface=on  Latency=0  AutoFrameSizeCalculation=off
  r x v : matrix_library/Cross Product
  r^2 : DotProduct  OutDataTypeStr=Inherit: Inherit via internal rule
  rate : Outport
  wires:
  R/1 -> r x v/1, r^2/2, r^2/1
  r x v/1 -> protected Division1/2
  r^2/1 -> protected Division1/1
  protected Division1/1 -> rate/1
  dR/1 -> r x v/2

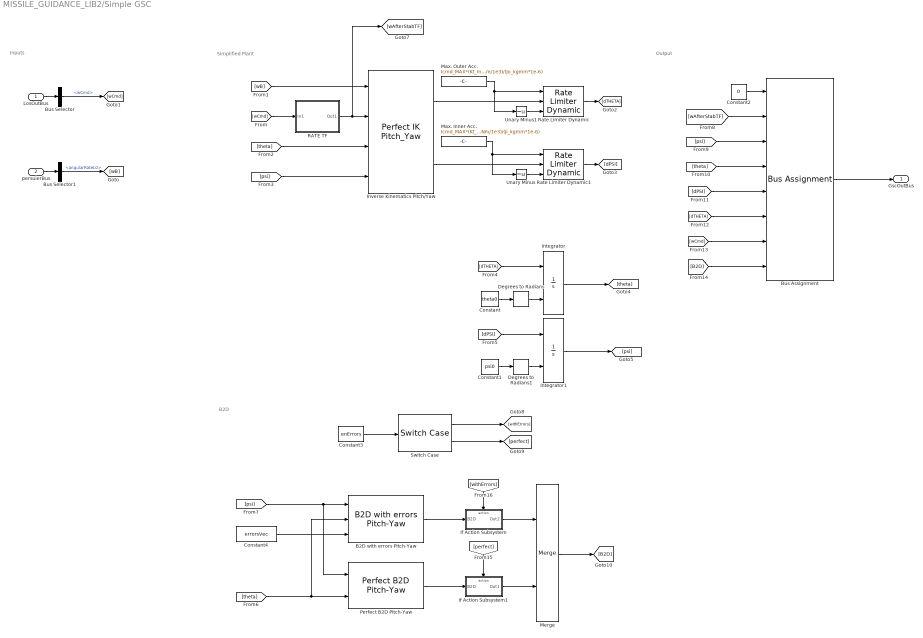
== system MISSILE_GUIDANCE_LIB2/Simple GSC ==
  note: B2D
  note: Output
  note: Simplified Plant
  note: Inputs
  LosOutBus : Inport  OutDataTypeStr=Bus: LosOutBus
  persuierBus : Inport  Port=2  OutDataTypeStr=Bus: missileBus
  B2D with errors Pitch-Yaw : $bdroot/B2D with errors Pitch-Yaw  SystemSampleTime=-1  VariantActivationTime=update diagram  AllowFlexibleInterface=on  Latency=0  AutoFrameSizeCalculation=off
  Bus Assignment : BusAssignment  AssignedSignals=wAfterStabTF,psiMeas,thetaMeas,psiDotCmd,thetaDotCmd,wCmd_Rtn,B2D
  Bus Selector : BusSelector  OutputSignals=wCmd
  Bus Selector1 : BusSelector  OutputSignals=angularRateL0
  Constant : Constant  Value=theta0
  Constant1 : Constant  Value=psi0
  Constant2 : Constant  Value=0  OutDataTypeStr=Bus: GscOutBus
  Constant3 : Constant  Value=enErrors
  Constant4 : Constant  Value=errorsVec
  Degrees to Radians : simulink_extras/Transformations/Degrees to Radians
  Degrees to Radians1 : simulink_extras/Transformations/Degrees to Radians
  If Action Subsystem : Subsystem  TreatAsAtomicUnit=on
  If Action Subsystem1 : Subsystem  TreatAsAtomicUnit=on
  Integrator : Integrator  InitialConditionSource=external
  Integrator1 : Integrator  InitialConditionSource=external
  Inverse Kinematics Pitch/Yaw : $bdroot/Perfect IK Pitch_Yaw  SystemSampleTime=-1  VariantActivationTime=update diagram  AllowFlexibleInterface=on  Latency=0  AutoFrameSizeCalculation=off
  Max. Inner Acc. : Constant  Value=Icmd_MAX*(Kt_mNm/1e3)/(Ji_kgmm*1e-6)
  Max. Outer Acc. : Constant  Value=Icmd_MAX*(Kt_mNm/1e3)/(Jo_kgmm*1e-6)
  Merge : Merge
  Perfect B2D Pitch-Yaw : $bdroot/Perfect B2D Pitch-Yaw  SystemSampleTime=-1  VariantActivationTime=update diagram  AllowFlexibleInterface=on  Latency=0  AutoFrameSizeCalculation=off
  RATE TF : Subsystem
  Rate Limiter Dynamic : simulink/Discontinuities/Rate Limiter Dynamic
  Rate Limiter Dynamic1 : simulink/Discontinuities/Rate Limiter Dynamic
  Switch Case : SwitchCase  CaseConditions={1, 0}  ShowDefaultCase=off
  Unary Minus : UnaryMinus
  Unary Minus1 : UnaryMinus
  GscOutBus : Outport  OutDataTypeStr=Bus: GscOutBus  SampleTime=1/f_clock_GSC
  wires:
  LosOutBus/1 -> Bus Selector/1
  persuierBus/1 -> Bus Selector1/1
  Bus Selector/1 -> [wCmd]  "<wCmd>"
  Bus Selector1/1 -> [wB]  "<angularRateL0>"
  [wCmd] -> RATE TF/1(In1)
  [wB] -> Inverse Kinematics Pitch/Yaw/1
  Inverse Kinematics Pitch/Yaw/1 -> Rate Limiter Dynamic/2
  [theta] -> Inverse Kinematics Pitch/Yaw/3
  [psi] -> Inverse Kinematics Pitch/Yaw/4
  Inverse Kinematics Pitch/Yaw/2 -> Rate Limiter Dynamic1/2
  [dTHETA] -> Integrator/1
  Constant/1 -> Degrees to Radians/1
  Degrees to Radians/1 -> Integrator/2
  Integrator/1 -> [theta]
  Constant1/1 -> Degrees to Radians1/1
  Integrator1/1 -> [psi]
  [dPSI] -> Integrator1/1
  Degrees to Radians1/1 -> Integrator1/2
  Constant2/1 -> Bus Assignment/1
  [wAfterStabTF] -> Bus Assignment/2
  [psi] -> Bus Assignment/3
  [theta] -> Bus Assignment/4
  [dPSI] -> Bus Assignment/5
  [dTHETA] -> Bus Assignment/6
  [wCmd] -> Bus Assignment/7
  [B2D] -> Bus Assignment/8
  RATE TF/1(Out1) -> [wAfterStabTF], Inverse Kinematics Pitch/Yaw/2
  Bus Assignment/1 -> GscOutBus/1
  Constant3/1 -> Switch Case/1
  Switch Case/1 -> [withErrors]
  Switch Case/2 -> [perfect]
  [withErrors] -> If Action Subsystem/Action
  [psi] -> Perfect B2D Pitch-Yaw/1, B2D with errors Pitch-Yaw/1
  [perfect] -> If Action Subsystem1/Action
  If Action Subsystem1/1(Out1) -> Merge/2
  If Action Subsystem/1(Out1) -> Merge/1
  Merge/1 -> [B2D]
  Perfect B2D Pitch-Yaw/1 -> If Action Subsystem1/1(B2D)
  B2D with errors Pitch-Yaw/1 -> If Action Subsystem/1(B2D)
  [theta] -> B2D with errors Pitch-Yaw/2, Perfect B2D Pitch-Yaw/2
  Constant4/1 -> B2D with errors Pitch-Yaw/3
  Rate Limiter Dynamic/1 -> [dTHETA]
  Rate Limiter Dynamic1/1 -> [dPSI]
  Max. Inner Acc./1 -> Unary Minus/1, Rate Limiter Dynamic1/1
  Unary Minus/1 -> Rate Limiter Dynamic1/3
  Max. Outer Acc./1 -> Rate Limiter Dynamic/1, Unary Minus1/1
  Unary Minus1/1 -> Rate Limiter Dynamic/3

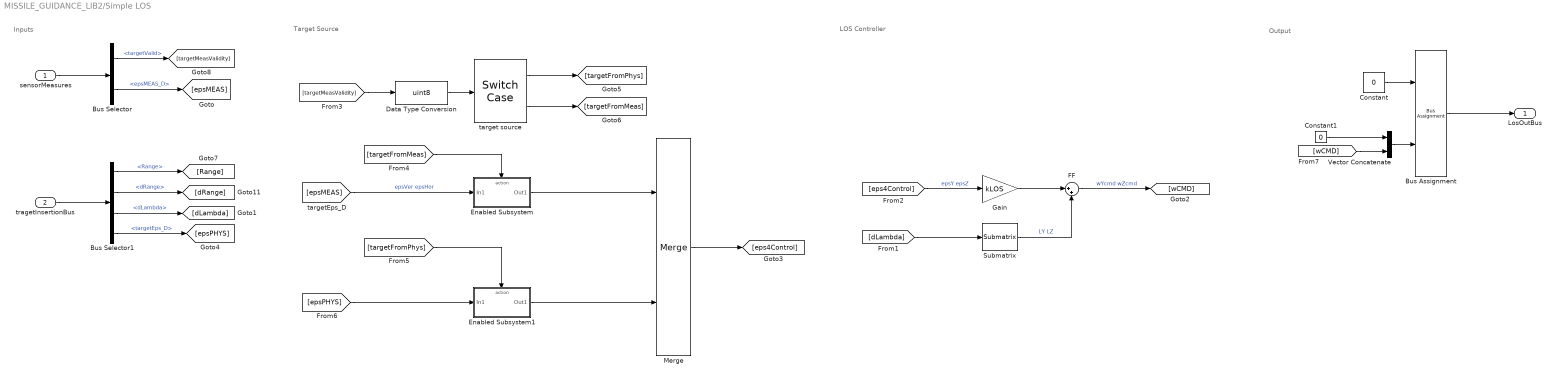
== system MISSILE_GUIDANCE_LIB2/Simple LOS ==
  note: LOS Controller
  note: Target Source
  note: Output
  note: Inputs
  sensorMeasures : Inport  OutDataTypeStr=Bus: sensorOutBus
  tragetInsertionBus : Inport  Port=2  OutDataTypeStr=Bus: targetInsertionBus
  Bus Assignment : BusAssignment  AssignedSignals=wCmd
  Bus Selector : BusSelector  OutputSignals=targetValid,epsMEAS_D
  Bus Selector1 : BusSelector  OutputSignals=Range,dRange,dLambda,targetEps_D
  Constant : Constant  Value=0  OutDataTypeStr=Bus: LosOutBus
  Constant1 : Constant  Value=0
  Data Type Conversion : DataTypeConversion  OutDataTypeStr=uint8  SaturateOnIntegerOverflow=off  RndMeth=Floor
  Enabled Subsystem : Subsystem  TreatAsAtomicUnit=on
  Enabled Subsystem1 : Subsystem  TreatAsAtomicUnit=on
  FF : Sum  Inputs=|++
  Gain : Gain  Gain=kLOS
  Merge : Merge
  Submatrix : matrix_library/Submatrix  RowSpan=Range of rows  RowStartMode=Index  RowStartIndex=2  RowEndMode=Last  RowEndIndex=1  ColSpan=All columns  ColStartMode=First  ColStartIndex=1  ColEndMode=Last  ColEndIndex=1
  Vector Concatenate : Concatenate
  target source : SwitchCase  CaseConditions={0,1}  ShowDefaultCase=off
  LosOutBus : Outport  OutDataTypeStr=Bus: LosOutBus  SampleTime=1/f_clock_LOS
  wires:
  sensorMeasures/1 -> Bus Selector/1
  Bus Selector/1 -> [targetMeasValidity]  "<targetValid>"
  tragetInsertionBus/1 -> Bus Selector1/1
  Bus Selector1/2 -> [dRange]  "<dRange>"
  Bus Selector1/1 -> [Range]  "<Range>"
  Bus Selector1/3 -> [dLambda]  "<dLambda>"
  [epsMEAS] -> Enabled Subsystem/1(In1)  "epsVer epsHor"
  Gain/1 -> FF/1
  Submatrix/1 -> FF/2  "LY LZ"
  [dLambda] -> Submatrix/1
  FF/1 -> [wCMD]  "wYcmd wZcmd"
  Bus Assignment/1 -> LosOutBus/1
  Constant/1 -> Bus Assignment/1
  [eps4Control] -> Gain/1  "epsY epsZ"
  [targetMeasValidity] -> Data Type Conversion/1
  target source/1 -> [targetFromPhys]
  target source/2 -> [targetFromMeas]
  [targetFromMeas] -> Enabled Subsystem/Action
  Enabled Subsystem/1(Out1) -> Merge/1
  Merge/1 -> [eps4Control]
  [epsPHYS] -> Enabled Subsystem1/1(In1)
  [targetFromPhys] -> Enabled Subsystem1/Action
  Enabled Subsystem1/1(Out1) -> Merge/2
  [wCMD] -> Vector Concatenate/2
  Vector Concatenate/1 -> Bus Assignment/2
  Constant1/1 -> Vector Concatenate/1
  Data Type Conversion/1 -> target source/1
  Bus Selector1/4 -> [epsPHYS]  "<targetEps_D>"
  Bus Selector/2 -> [epsMEAS]  "<epsMEAS_D>"

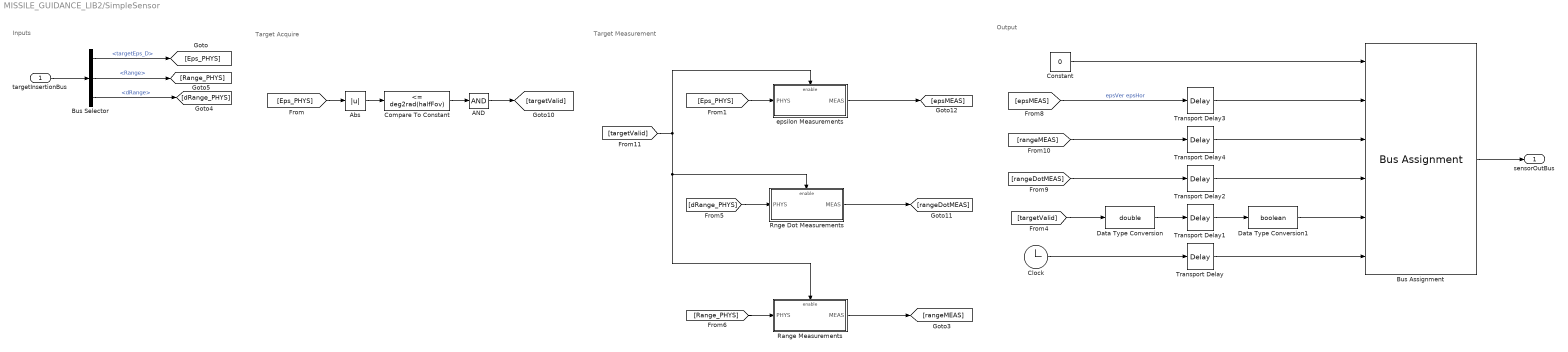
== system MISSILE_GUIDANCE_LIB2/SimpleSensor ==
  note: Target Measurement
  note: Target Acquire
  note: Output
  note: Inputs
  targetInsertionBus : Inport  OutDataTypeStr=Bus: targetInsertionBus
  AND : Logic  Inputs=1  AllPortsSameDT=off  OutDataTypeStr=boolean
  Abs : Abs  SaturateOnIntegerOverflow=off
  Bus Assignment : BusAssignment  AssignedSignals=epsMEAS_D,rangeMEAS_D,rangeDotMEAS_D,targetValid,timeOfMeas
  Bus Selector : BusSelector  OutputSignals=targetEps_D,Range,dRange
  Clock : Clock
  Compare To Constant : simulink/Logic and Bit Operations/Compare To Constant  relop=<=  const=deg2rad(halfFov)  OutDataTypeStr=boolean
  Constant : Constant  Value=0  OutDataTypeStr=Bus: sensorOutBus
  Data Type Conversion : DataTypeConversion  OutDataTypeStr=double  SaturateOnIntegerOverflow=off  RndMeth=Floor
  Data Type Conversion1 : DataTypeConversion  OutDataTypeStr=boolean  SaturateOnIntegerOverflow=off  RndMeth=Floor
  Range Measurements : Subsystem
  Rnge Dot Measurements : Subsystem
  Transport Delay{,1..4} (5 alike) : TransportDelay  DelayTime=tLatency*1e-3  PadeOrder=2
  epsilon Measurements : Subsystem
  sensorOutBus : Outport  OutDataTypeStr=Bus: sensorOutBus  SampleTime=1/f_clock_SENS
  wires:
  targetInsertionBus/1 -> Bus Selector/1
  Constant/1 -> Bus Assignment/1
  Bus Selector/1 -> [Eps_PHYS]  "<targetEps_D>"
  Bus Selector/3 -> [dRange_PHYS]  "<dRange>"
  Bus Selector/2 -> [Range_PHYS]  "<Range>"
  [Eps_PHYS] -> Abs/1
  Abs/1 -> Compare To Constant/1
  Compare To Constant/1 -> AND/1
  [dRange_PHYS] -> Rnge Dot Measurements/1(PHYS)
  [Range_PHYS] -> Range Measurements/1(PHYS)
  [Eps_PHYS] -> epsilon Measurements/1(PHYS)
  [epsMEAS] -> Transport Delay3/1  "epsVer epsHor"
  [rangeDotMEAS] -> Transport Delay2/1
  [rangeMEAS] -> Transport Delay4/1
  AND/1 -> [targetValid]
  [targetValid] -> Range Measurements/Enable, Rnge Dot Measurements/Enable, epsilon Measurements/Enable
  Range Measurements/1(MEAS) -> [rangeMEAS]
  Rnge Dot Measurements/1(MEAS) -> [rangeDotMEAS]
  epsilon Measurements/1(MEAS) -> [epsMEAS]
  [targetValid] -> Data Type Conversion/1
  Bus Assignment/1 -> sensorOutBus/1
  Clock/1 -> Transport Delay/1
  Transport Delay/1 -> Bus Assignment/6
  Transport Delay1/1 -> Data Type Conversion1/1
  Transport Delay2/1 -> Bus Assignment/4
  Transport Delay3/1 -> Bus Assignment/2
  Transport Delay4/1 -> Bus Assignment/3
  Data Type Conversion/1 -> Transport Delay1/1
  Data Type Conversion1/1 -> Bus Assignment/5

== system MISSILE_GUIDANCE_LIB2/Simulation Stop ==
  targetInsertionBus : Inport  OutDataTypeStr=Bus: targetInsertionBus
  Bus Selector : BusSelector  OutputSignals=t_go
  Compare To Constant : simulink/Logic and Bit Operations/Compare To Constant  relop=<=  const=0  OutDataTypeStr=boolean
  Stop Simulation : Stop
  wires:
  targetInsertionBus/1 -> Bus Selector/1
  Bus Selector/1 -> Compare To Constant/1  "<t_go>"
  Compare To Constant/1 -> Stop Simulation/1
